simulink model "fluids_and_control"  (R2024b)
settings: Solver=VariableStepAuto  StartTime=0.0  StopTime=stopTime  RelTol=1e-3
settings Model: SimulationMode=rapid-accelerator  TunableVars=AC_tank_cross_sectional_area,AC_tank_radius,AC_tank_surface_area,AC_tank_vol_limit,AC_tank_volume,AC_tank_weight,AC_wall_thickness,Ambient_temp,Equivalent_battery_mass,GH2_conductivity,Generator_efficiency,H2Tables,H2_energy_density,Initial_AC_LH2_frac,Initial_AC_Tank_Gas_Temp,Initial_AC_Tank_Liquid_Temp,Initial_AC_tank_pressure,Initial_temp,LH2_conductivity,LH2_density,LH2_density_table,Required_energy,Temp_vector,engine_feed_pipe_inner_area,engine_feed_pipe_inner_diameter,engine_feed_pipe_outer_area,engine_feed_pipe_outer_diameter,engine_feed_valve_discharge_ratio,engine_feed_valve_orifice_area,engine_feed_valve_orifice_radius,hose_length,hose_thermal_conductivity,initial_hose_p,liquid_supply_SOV_leak_frac,m_LH2,mass_flow_rate,mass_per_length_engine_feed,mass_per_length_return,mass_per_length_supply,max_pressure,max_stress,phase,pipe_thermal_conductivity,pressure_vector,radiation_constant,refuel_time,return_pipe_inner_area,return_pipe_inner_diameter,return_pipe_outer_area,return_pipe_outer_diameter,return_valve_discharge_ratio,return_valve_orifice_area,return_valve_orifice_radius,short_pressure_vector,short_temp_vector,steel_conductivity,steel_density,steel_emmissitivity,steel_heat_capacity,stopTime,supply_pipe_inner_area,supply_pipe_inner_diameter,supply_pipe_outer_area,supply_pipe_outer_diameter,supply_valve_discharge_ratio,supply_valve_orifice_area,supply_valve_orifice_radius,timestep,u_max_gas,u_min_liquid,wall_thickness,valve_laminar_p_ratio  TunableVarsStorageClass=Auto,Auto,Auto,Auto,Auto,Auto,Auto,Auto,Auto,Auto,Auto,Auto,Auto,Auto,Auto,Auto,Auto,Auto,Auto,Auto,Auto,Auto,Auto,Auto,Auto,Auto,Auto,Auto,Auto,Auto,Auto,Auto,Auto,Auto,Auto,Auto,Auto,Auto,Auto,Auto,Auto,Auto,Auto,Auto,Auto,Auto,Auto,Auto,Auto,Auto,Auto,Auto,Auto,Auto,Auto,Auto,Auto,Auto,Auto,Auto,Auto,Auto,Auto,Auto,Auto,Auto,Auto,Auto,Auto,Auto,Auto,Auto  TunableVarsTypeQualifier=,,,,,,,,,,,,,,,,,,,,,,,,,,,,,,,,,,,,,,,,,,,,,,,,,,,,,,,,,,,,,,,,,,,,,,,  Creator=MW  LastModifiedBy=MW

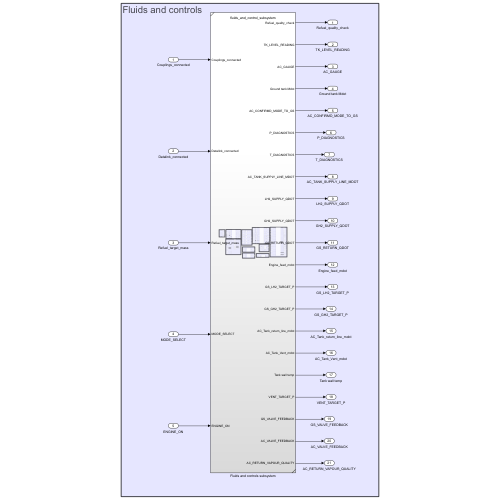
[thumbnail: Simulink's stored preview of the top-level diagram]
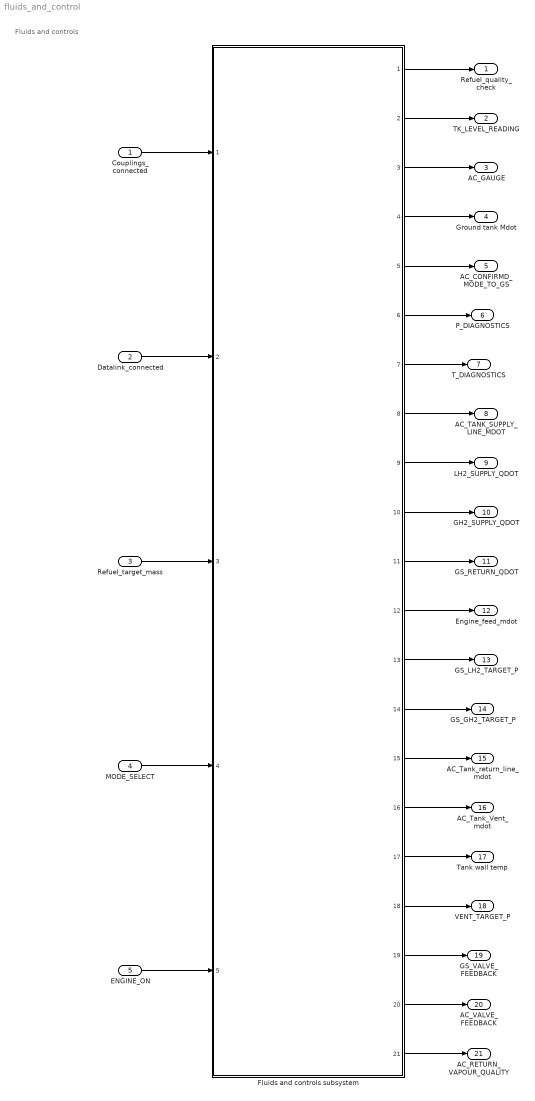
== system fluids_and_control ==
  note: Fluids and controls
  Couplings_connected : Inport
  Datalink_connected : Inport  Port=2
  Refuel_target_mass : Inport  Port=3
  MODE_SELECT : Inport  Port=4
  ENGINE_ON : Inport  Port=5
  Fluids and controls subsystem : Subsystem  ReferencedSubsystem=fluids_and_control_subsystem
  Refuel_quality_check : Outport
  TK_LEVEL_READING : Outport  Port=2
  AC_GAUGE : Outport  Port=3
  Ground tank Mdot : Outport  Port=4
  AC_CONFIRMD_MODE_TO_GS : Outport  Port=5
  P_DIAGNOSTICS : Outport  Port=6
  T_DIAGNOSTICS : Outport  Port=7
  AC_TANK_SUPPLY_LINE_MDOT : Outport  Port=8
  LH2_SUPPLY_QDOT : Outport  Port=9
  GH2_SUPPLY_QDOT : Outport  Port=10
  GS_RETURN_QDOT : Outport  Port=11
  Engine_feed_mdot : Outport  Port=12
  GS_LH2_TARGET_P : Outport  Port=13
  GS_GH2_TARGET_P : Outport  Port=14
  AC_Tank_return_line_mdot : Outport  Port=15
  AC_Tank_Vent_mdot : Outport  Port=16
  Tank wall temp : Outport  Port=17
  VENT_TARGET_P : Outport  Port=18
  GS_VALVE_FEEDBACK : Outport  Port=19
  AC_VALVE_FEEDBACK : Outport  Port=20
  AC_RETURN_VAPOUR_QUALITY : Outport  Port=21
  wires:
  Fluids and controls subsystem/6 -> P_DIAGNOSTICS/1
  Fluids and controls subsystem/16 -> AC_Tank_Vent_mdot/1
  Fluids and controls subsystem/3 -> AC_GAUGE/1
  Datalink_connected/1 -> Fluids and controls subsystem/2
  Fluids and controls subsystem/9 -> LH2_SUPPLY_QDOT/1
  Fluids and controls subsystem/11 -> GS_RETURN_QDOT/1
  Fluids and controls subsystem/2 -> TK_LEVEL_READING/1
  Fluids and controls subsystem/5 -> AC_CONFIRMD_MODE_TO_GS/1
  Fluids and controls subsystem/1 -> Refuel_quality_check/1
  Fluids and controls subsystem/14 -> GS_GH2_TARGET_P/1
  Fluids and controls subsystem/17 -> Tank wall temp/1
  Refuel_target_mass/1 -> Fluids and controls subsystem/3
  Fluids and controls subsystem/13 -> GS_LH2_TARGET_P/1
  Couplings_connected/1 -> Fluids and controls subsystem/1
  ENGINE_ON/1 -> Fluids and controls subsystem/5
  Fluids and controls subsystem/19 -> GS_VALVE_FEEDBACK/1
  Fluids and controls subsystem/10 -> GH2_SUPPLY_QDOT/1
  Fluids and controls subsystem/8 -> AC_TANK_SUPPLY_LINE_MDOT/1
  Fluids and controls subsystem/7 -> T_DIAGNOSTICS/1
  Fluids and controls subsystem/12 -> Engine_feed_mdot/1
  MODE_SELECT/1 -> Fluids and controls subsystem/4
  Fluids and controls subsystem/15 -> AC_Tank_return_line_mdot/1
  Fluids and controls subsystem/4 -> Ground tank Mdot/1
  Fluids and controls subsystem/18 -> VENT_TARGET_P/1
  Fluids and controls subsystem/20 -> AC_VALVE_FEEDBACK/1
  Fluids and controls subsystem/21 -> AC_RETURN_VAPOUR_QUALITY/1
